simulink model "matrixmul_sysgen_cosim"  (R2017a)
settings: Solver=VariableStepAuto  StartTime=0.0  StopTime=45  RelTol=1e-3
values from neighbouring files (symbols this model uses):
  A = [1 2 8 4; 5 2 7 0; 9 10 4 2; 7 0 3 1]    [loadmatrix.m]
undefined symbols (not defined in the file or in its folder): N
libraries: xbsIndex_r4 x26, JTAGRuntimeCosim_r4 x1
settings Model: Creator=jhell  LastModifiedBy=jlh24

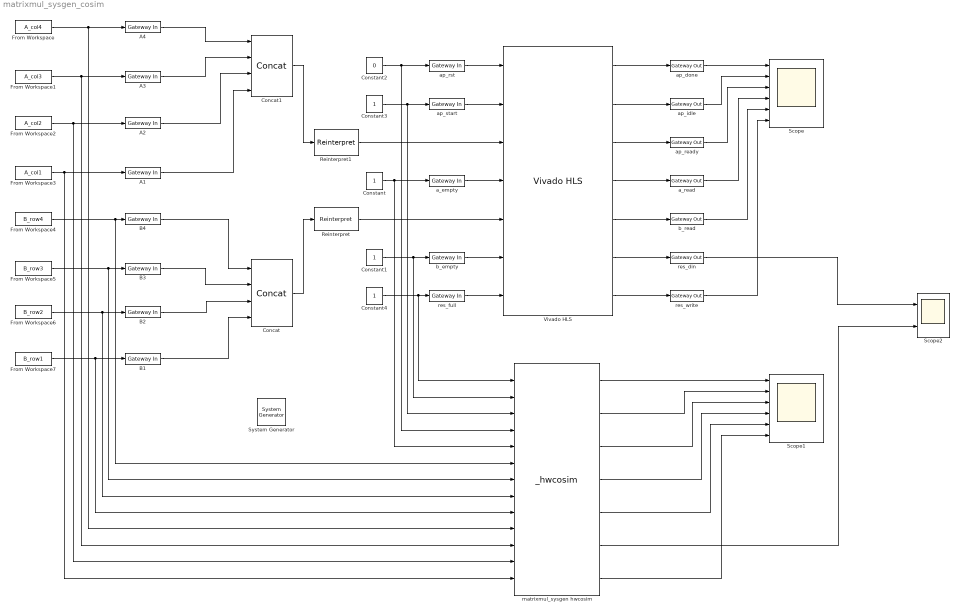
== system matrixmul_sysgen_cosim ==
  " System Generator" : xbsIndex_r4/ System Generator  Tag=genX  xilinxfamily=zynq  part=xc7z020  speed=-1  package=clg484  synthesis_tool=Vivado  clock_wrapper=Clock Enables  directory=./netlist_cosim  proj_type=Vivado  Synth_file=Vivado Synthesis Defaults  Impl_file=Vivado Implementation Defaults  testbench=off  simulink_period=1  sysclk_period=10  dcm_input_clock_period=10  incr_netlist=off  trim_vbits=Everywhere in SubSystem  dbl_ovrd=According to Block Masks  core_generation=According to Block Masks  run_coregen=off  deprecated_control=off  eval_field=0  block_type=sysgen
  A{1..4} (4 alike) : xbsIndex_r4/Gateway In  gui_display_data_type=Fixed-point  arith_type=Unsigned  n_bits=16  bin_pt=0  preci_type=Single  exp_width=8  frac_width=24  rows=1  columns=1  quantization="Round  (unbiased: +/- Inf)"  overflow=Saturate  period=1  UseAsADC=off  ADCChannel='1'  interface=None  automatic_assignment=on  address_offset=hex2dec('00')  intf_name=''  intf_description=''  default_value=0  timing_constraint=None  locs_specified=off  LOCs={}  io_standard={}  inherit_from_input=off  hdl_port=on  dbl_ovrd=off  block_type=gatewayin
  B{1..4} (4 alike) : xbsIndex_r4/Gateway In  gui_display_data_type=Fixed-point  arith_type=Unsigned  n_bits=16  bin_pt=0  preci_type=Single  exp_width=8  frac_width=24  rows=1  columns=1  quantization="Round  (unbiased: +/- Inf)"  overflow=Saturate  period=1  UseAsADC=off  ADCChannel='1'  interface=None  automatic_assignment=on  address_offset=hex2dec('00')  intf_name=''  intf_description=''  default_value=0  timing_constraint=None  locs_specified=off  LOCs={}  io_standard={}  inherit_from_input=off  hdl_port=on  dbl_ovrd=off  block_type=gatewayin
  Concat : xbsIndex_r4/Concat  num_inputs=4  dbl_ovrd=off  block_type=concat
  Concat1 : xbsIndex_r4/Concat  num_inputs=4  dbl_ovrd=off  block_type=concat
  Constant{,1,3..4} (4 alike) : Constant
  Constant2 : Constant  Value=0
  From Workspace : FromWorkspace  VariableName=A_col4  SampleTime=0  Interpolate=off  OutputAfterFinalValue=Setting to zero
  From Workspace1 : FromWorkspace  VariableName=A_col3  SampleTime=0  Interpolate=off  OutputAfterFinalValue=Setting to zero
  From Workspace2 : FromWorkspace  VariableName=A_col2  SampleTime=0  Interpolate=off  OutputAfterFinalValue=Setting to zero
  From Workspace3 : FromWorkspace  VariableName=A_col1  SampleTime=0  Interpolate=off  OutputAfterFinalValue=Setting to zero
  From Workspace4 : FromWorkspace  VariableName=B_row4  SampleTime=0  Interpolate=off  OutputAfterFinalValue=Setting to zero
  From Workspace5 : FromWorkspace  VariableName=B_row3  SampleTime=0  Interpolate=off  OutputAfterFinalValue=Setting to zero
  From Workspace6 : FromWorkspace  VariableName=B_row2  SampleTime=0  Interpolate=off  OutputAfterFinalValue=Setting to zero
  From Workspace7 : FromWorkspace  VariableName=B_row1  SampleTime=0  Interpolate=off  OutputAfterFinalValue=Setting to zero
  Reinterpret : xbsIndex_r4/Reinterpret  force_arith_type=on  arith_type="Signed  (2's comp)"  force_bin_pt=off  bin_pt=0  block_type=reinterpret
  Reinterpret1 : xbsIndex_r4/Reinterpret  force_arith_type=on  arith_type="Signed  (2's comp)"  force_bin_pt=off  bin_pt=0  block_type=reinterpret
  Scope : Scope  NumInputPorts=6
  Scope1 : Scope  NumInputPorts=6
  Scope2 : Scope  NumInputPorts=2
  Vivado HLS : xbsIndex_r4/Vivado HLS  anytable='C:/ELEC522/hellar/Project_3/matrixmul_final/matrixmul_final/solution1'  fast_sim=off  display_datatype=on  rate_propagation_method=Simulink system period  model_file_path=''  latency=1  block_type=hls
      settings: infoedit=This block allows including C,C++ and SystemC source files in System Generator for DSP designs.
  a_empty : xbsIndex_r4/Gateway In  gui_display_data_type=Boolean  arith_type=Boolean  n_bits=16  bin_pt=14  preci_type=Single  exp_width=8  frac_width=24  rows=1  columns=1  quantization="Round  (unbiased: +/- Inf)"  overflow=Saturate  period=1  UseAsADC=off  ADCChannel='1'  interface=None  automatic_assignment=on  address_offset=hex2dec('00')  intf_name=''  intf_description=''  default_value=0  timing_constraint=None  locs_specified=off  LOCs={}  io_standard={}  inherit_from_input=off  hdl_port=on  dbl_ovrd=off  block_type=gatewayin
  a_read : xbsIndex_r4/Gateway Out  inherit_from_input=off  hdl_port=on  rows=1  columns=1  UseAsDAC=off  DACChannel='1'  interface=None  automatic_assignment=on  address_offset=hex2dec('00')  intf_name=''  intf_description=''  timing_constraint=None  locs_specified=off  LOCs={}  io_standard={}  block_type=gatewayout
  ap_done : xbsIndex_r4/Gateway Out  inherit_from_input=off  hdl_port=on  rows=1  columns=1  UseAsDAC=off  DACChannel='1'  interface=None  automatic_assignment=on  address_offset=hex2dec('00')  intf_name=''  intf_description=''  timing_constraint=None  locs_specified=off  LOCs={}  io_standard={}  block_type=gatewayout
  ap_idle : xbsIndex_r4/Gateway Out  inherit_from_input=off  hdl_port=on  rows=1  columns=1  UseAsDAC=off  DACChannel='1'  interface=None  automatic_assignment=on  address_offset=hex2dec('00')  intf_name=''  intf_description=''  timing_constraint=None  locs_specified=off  LOCs={}  io_standard={}  block_type=gatewayout
  ap_ready : xbsIndex_r4/Gateway Out  inherit_from_input=off  hdl_port=on  rows=1  columns=1  UseAsDAC=off  DACChannel='1'  interface=None  automatic_assignment=on  address_offset=hex2dec('00')  intf_name=''  intf_description=''  timing_constraint=None  locs_specified=off  LOCs={}  io_standard={}  block_type=gatewayout
  ap_rst : xbsIndex_r4/Gateway In  gui_display_data_type=Boolean  arith_type=Boolean  n_bits=16  bin_pt=14  preci_type=Single  exp_width=8  frac_width=24  rows=1  columns=1  quantization="Round  (unbiased: +/- Inf)"  overflow=Saturate  period=1  UseAsADC=off  ADCChannel='1'  interface=None  automatic_assignment=on  address_offset=hex2dec('00')  intf_name=''  intf_description=''  default_value=0  timing_constraint=None  locs_specified=off  LOCs={}  io_standard={}  inherit_from_input=off  hdl_port=on  dbl_ovrd=off  block_type=gatewayin
  ap_start : xbsIndex_r4/Gateway In  gui_display_data_type=Boolean  arith_type=Boolean  n_bits=16  bin_pt=14  preci_type=Single  exp_width=8  frac_width=24  rows=1  columns=1  quantization="Round  (unbiased: +/- Inf)"  overflow=Saturate  period=1  UseAsADC=off  ADCChannel='1'  interface=None  automatic_assignment=on  address_offset=hex2dec('00')  intf_name=''  intf_description=''  default_value=0  timing_constraint=None  locs_specified=off  LOCs={}  io_standard={}  inherit_from_input=off  hdl_port=on  dbl_ovrd=off  block_type=gatewayin
  b_empty : xbsIndex_r4/Gateway In  gui_display_data_type=Boolean  arith_type=Boolean  n_bits=16  bin_pt=14  preci_type=Single  exp_width=8  frac_width=24  rows=1  columns=1  quantization="Round  (unbiased: +/- Inf)"  overflow=Saturate  period=1  UseAsADC=off  ADCChannel='1'  interface=None  automatic_assignment=on  address_offset=hex2dec('00')  intf_name=''  intf_description=''  default_value=0  timing_constraint=None  locs_specified=off  LOCs={}  io_standard={}  inherit_from_input=off  hdl_port=on  dbl_ovrd=off  block_type=gatewayin
  b_read : xbsIndex_r4/Gateway Out  inherit_from_input=off  hdl_port=on  rows=1  columns=1  UseAsDAC=off  DACChannel='1'  interface=None  automatic_assignment=on  address_offset=hex2dec('00')  intf_name=''  intf_description=''  timing_constraint=None  locs_specified=off  LOCs={}  io_standard={}  block_type=gatewayout
  matrixmul_sysgen hwcosim : JTAGRuntimeCosim_r4/_hwcosim  clkSrc=Single Stepped  hasCombinationalPath=on  bitfileName=C:\ELEC522\hellar\Project_3\matrixmul_final\netlist_cosim\matrixmul_sysgen.bit  skipConfig=off  dispPartInfo=off  useZynqReconfigScript=on  cable=Auto Detect  speed=N/A  cablePort=N/A  cableLocation=Local  shareCable=off  design_xtable=|  engineDll=JTAGCosimEngine.dll  cableWaitTime=10  bscanPos=-1  IRLengths=[]  useWaitBox=1  hasBufgmux=on  Scheme=Cosim  useCmdProc=1  hasProc=0  useImpact=0  printLogFile=0  userChain=2  block_type=jtagcosim
      | {
      |     'clkWrapper' => 'matrixmul_sysgen',
      |     'burstMode' => false,
      |     'burstFifoDepth' => '1024',
      |     'shared_memories' => {},
      |     'clocksGcd' => 1,
      |     'device' => {
      |       'family' => 'zynq',
      |       'part' => 'xc7z020',
      |       'package' => 'clg484',
      |       'speed' => '-1',
      |     },
      |     'ports' => {
      |       'res_full' => {
      |         'direction' => 'in',
      |         'width' => 1,
      |         'name' => 'res_full',
      |         'period' => 1,
      |         'icon_text' => 'res_full',
      |         'type' => 'Bool',
      |         'arithmetic_type' => 'xlUnsigned',
      |         'dat_file' => 'matrixmul_sysgen_res_full.dat',
      |         'bin_pt' => 0,
      |         'addr_offset' => 0,
      |         'bd_port_index' => 0,
      |       },
      |       'b_empty' => {
      |         'direction' => 'in',
      |         'width' => 1,
      |         'name' => 'b_empty',
      |         'period' => 1,
      |         'icon_text' => 'b_empty',
      |         'type' => 'Bool',
      |         'arithmetic_type' => 'xlUnsigned',
      |         'dat_file' => 'matrixmul_sysgen_b_empty.dat',
      |         'bin_pt' => 0,
      |         'addr_offset' => 4,
      |         'bd_port_index' => 1,
      |       },
      |       'ap_start' => {
      |         'direction' => 'in',
      |         'width' => 1,
      |         'name' => 'ap_start',
      |         'period' => 1,
      |         'icon_text' => 'ap_start',
      |         'type' => 'Bool',
      |         'arithmetic_type' => 'xlUnsigned',
      |         'dat_file' => 'matrixmul_sysgen_ap_start.dat',
      |         'bin_pt' => 0,
      |         'addr_offset' => 8,
      |         'bd_port_index' => 2,
      |       },
      |       'ap_rst' => {
      |         'direction' => 'in',
      |         'width' => 1,
      |         'name' => 'ap_rst',
      |         'period' => 1,
      |         'icon_text' => 'ap_rst',
      |         'type' => 'Bool',
      |         'arithmetic_type' => 'xlUnsigned',
      |         'dat_file' => 'matrixmul_sysgen_ap_rst.dat',
      |         'bin_pt' => 0,
      |         'addr_offset' => 12,
      |         'bd_port_index' => 3,
      |       },
      |       'a_empty' => {
      |         'direction' => 'in',
      |         'width' => 1,
      |         'name' => 'a_empty',
      |         'period' => 1,
      |         'icon_text' => 'a_empty',
      |         'type' => 'Bool',
      |         'arithmetic_type' => 'xlUnsigned',
      |         'dat_file' => 'matrixmul_sysgen_a_empty.dat',
      |         'bin_pt' => 0,
      |         'addr_offset' => 16,
      |         'bd_port_index' => 4,
      |       },
      |       'b4' => {
      |         'direction' => 'in',
      |         'width' => 16,
      |         'name' => 'b4',
      |         'period' => 1,
      |         'icon_text' => 'B4',
      |         'type' => 'UFix_16_0',
      |         'arithmetic_type' => 'xlUnsigned',
      |         'dat_file' => 'matrixmul_sysgen_b4.dat',
      |         'bin_pt' => 0,
      |         'addr_offset' => 20,
      |         'bd_port_index' => 5,
      |       },
      |       'b3' => {
      |         'direction' => 'in',
      |         'width' => 16,
      |         'name' => 'b3',
      |         'period' => 1,
      |         'icon_text' => 'B3',
      |         'type' => 'UFix_16_0',
      |         'arithmetic_type' => 'xlUnsigned',
      |         'dat_file' => 'matrixmul_sysgen_b3.dat',
      |         'bin_pt' => 0,
      |         'addr_offset' => 24,
      |         'bd_port_index' => 6,
      |       },
      |       'b2' => {
      |         'direction' => 'in',
      |         'width' => 16,
      |         'name' => 'b2',
      |         'period' => 1,
      |         'icon_text' => 'B2',
      |         'type' => 'UFix_16_0',
      |         'arithmetic_type' => 'xlUnsigned',
      |         'dat_file' => 'matrixmul_sysgen_b2.dat',
      |         'bin_pt' => 0,
      |         'addr_offset' => 28,
      |         'bd_port_index' => 7,
      |       },
      |       'b1' => {
      |         'direction' => 'in',
      |         'width' => 16,
      |         'name' => 'b1',
      |         'period' => 1,
      |         'icon_text' => 'B1',
      |         'type' => 'UFix_16_0',
      |         'arithmetic_type' => 'xlUnsigned',
      |         'dat_file' => 'matrixmul_sysgen_b1.dat',
      |         'bin_pt' => 0,
      |         'addr_offset' => 32,
      |         'bd_port_index' => 8,
      |       },
      |       'a4' => {
      |         'direction' => 'in',
      |         'width' => 16,
      |         'name' => 'a4',
      |         'period' => 1,
      |         'icon_text' => 'A4',
      |         'type' => 'UFix_16_0',
      |         'arithmetic_type' => 'xlUnsigned',
      |         'dat_file' => 'matrixmul_sysgen_a4.dat',
      |         'bin_pt' => 0,
      |         'addr_offset' => 36,
      |         'bd_port_index' => 9,
      |       },
      |       'a3' => {
      |         'direction' => 'in',
      |         'width' => 16,
      |         'name' => 'a3',
      |         'period' => 1,
      |         'icon_text' => 'A3',
      |         'type' => 'UFix_16_0',
      |         'arithmetic_type' => 'xlUnsigned',
      |         'dat_file' => 'matrixmul_sysgen_a3.dat',
      |         'bin_pt' => 0,
      |         'addr_offset' => 40,
      |         'bd_port_index' => 10,
      |       },
      |       'a2' => {
      |         'direction' => 'in',
      |         'width' => 16,
      |         'name' => 'a2',
      |         'period' => 1,
      |         'icon_text' => 'A2',
      |         'type' => 'UFix_16_0',
      |         'arithmetic_type' => 'xlUnsigned',
      |         'dat_file' => 'matrixmul_sysgen_a2.dat',
      |         'bin_pt' => 0,
      |         'addr_offset' => 44,
      |         'bd_port_index' => 11,
      |       },
      |       'a1' => {
      |         'direction' => 'in',
      |         'width' => 16,
      |         'name' => 'a1',
      |         'period' => 1,
      |         'icon_text' => 'A1',
      |         'type' => 'UFix_16_0',
      |         'arithmetic_type' => 'xlUnsigned',
      |         'dat_file' => 'matrixmul_sysgen_a1.dat',
      |         'bin_pt' => 0,
      |         'addr_offset' => 48,
      |         'bd_port_index' => 12,
      |       },
      |       'a_read' => {
      |         'direction' => 'out',
      |         'width' => 1,
      |         'name' => 'a_read',
      |         'period' => 1,
      |         'icon_text' => 'a_read',
      |         'type' => 'Bool',
      |         'arithmetic_type' => 'xlUnsigned',
      |         'dat_file' => 'matrixmul_sysgen_a_read.dat',
      |         'bin_pt' => 0,
      |         'addr_offset' => 52,
      |         'bd_port_index' => 0,
      |       },
      |       'ap_done' => {
      |         'direction' => 'out',
      |         'width' => 1,
      |         'name' => 'ap_done',
      |         'period' => 1,
      |         'icon_text' => 'ap_done',
      |         'type' => 'Bool',
      |         'arithmetic_type' => 'xlUnsigned',
      |         'dat_file' => 'matrixmul_sysgen_ap_done.dat',
      |         'bin_pt' => 0,
      |         'addr_offset' => 56,
      |         'bd_port_index' => 1,
      |       },
      |       'ap_idle' => {
      |         'direction' => 'out',
      |         'width' => 1,
      |         'name' => 'ap_idle',
      |         'period' => 1,
      |         'icon_text' => 'ap_idle',
      |         'type' => 'Bool',
      |         'arithmetic_type' => 'xlUnsigned',
      |         'dat_file' => 'matrixmul_sysgen_ap_idle.dat',
      |         'bin_pt' => 0,
      |         'addr_offset' => 60,
      |         'bd_port_index' => 2,
      |       },
      |       'ap_ready' => {
      |         'direction' => 'out',
      |         'width' => 1,
      |         'name' => 'ap_ready',
      |         'period' => 1,
      |         'icon_text' => 'ap_ready',
      |         'type' => 'Bool',
      |         'arithmetic_type' => 'xlUnsigned',
      |         'dat_file' => 'matrixmul_sysgen_ap_ready.dat',
      |         'bin_pt' => 0,
      |         'addr_offset' => 64,
      |         'bd_port_index' => 3,
      |       },
      |       'b_read' => {
      |         'direction' => 'out',
      |         'width' => 1,
      |         'name' => 'b_read',
      |         'period' => 1,
      |         'icon_text' => 'b_read',
      |         'type' => 'Bool',
      |         'arithmetic_type' => 'xlUnsigned',
      |         'dat_file' => 'matrixmul_sysgen_b_read.dat',
      |         'bin_pt' => 0,
      |         'addr_offset' => 68,
      |         'bd_port_index' => 4,
      |       },
      |       'res_din' => {
      |         'direction' => 'out',
      |         'width' => 16,
      |         'name' => 'res_din',
      |         'period' => 1,
      |         'icon_text' => 'res_din',
      |         'type' => 'Fix_16_0',
      |         'arithmetic_type' => 'xlSigned',
      |         'dat_file' => 'matrixmul_sysgen_res_din.dat',
      |         'bin_pt' => 0,
      |         'addr_offset' => 72,
      |         'bd_port_index' => 5,
      |       },
      |       'res_write' => {
      |         'direction' => 'out',
      |         'width' => 1,
      |         'name' => 'res_write',
      |         'period' => 1,
      |         'icon_text' => 'res_write',
      |         'type' => 'Bool',
      |         'arithmetic_type' => 'xlUnsigned',
      |         'dat_file' => 'matrixmul_sysgen_res_write.dat',
      |         'bin_pt' => 0,
      |         'addr_offset' => 76,
      |         'bd_port_index' => 6,
      |       },
      |     },
      |   }
  res_din : xbsIndex_r4/Gateway Out  inherit_from_input=off  hdl_port=on  rows=1  columns=1  UseAsDAC=off  DACChannel='1'  interface=None  automatic_assignment=on  address_offset=hex2dec('00')  intf_name=''  intf_description=''  timing_constraint=None  locs_specified=off  LOCs={}  io_standard={}  block_type=gatewayout
  res_full : xbsIndex_r4/Gateway In  gui_display_data_type=Boolean  arith_type=Boolean  n_bits=16  bin_pt=14  preci_type=Single  exp_width=8  frac_width=24  rows=1  columns=1  quantization="Round  (unbiased: +/- Inf)"  overflow=Saturate  period=1  UseAsADC=off  ADCChannel='1'  interface=None  automatic_assignment=on  address_offset=hex2dec('00')  intf_name=''  intf_description=''  default_value=0  timing_constraint=None  locs_specified=off  LOCs={}  io_standard={}  inherit_from_input=off  hdl_port=on  dbl_ovrd=off  block_type=gatewayin
  res_write : xbsIndex_r4/Gateway Out  inherit_from_input=off  hdl_port=on  rows=1  columns=1  UseAsDAC=off  DACChannel='1'  interface=None  automatic_assignment=on  address_offset=hex2dec('00')  intf_name=''  intf_description=''  timing_constraint=None  locs_specified=off  LOCs={}  io_standard={}  block_type=gatewayout
  wires:
  ap_start/1 -> Vivado HLS/2
  a_empty/1 -> Vivado HLS/4
  Constant3/1 -> matrixmul_sysgen hwcosim/3, ap_start/1
  Constant/1 -> matrixmul_sysgen hwcosim/5, a_empty/1
  Constant1/1 -> matrixmul_sysgen hwcosim/2, b_empty/1
  b_empty/1 -> Vivado HLS/6
  res_full/1 -> Vivado HLS/7
  Reinterpret/1 -> Vivado HLS/5
  Concat/1 -> Reinterpret/1
  Concat1/1 -> Reinterpret1/1
  A4/1 -> Concat1/1
  A3/1 -> Concat1/2
  A2/1 -> Concat1/3
  A1/1 -> Concat1/4
  B4/1 -> Concat/1
  B3/1 -> Concat/2
  B2/1 -> Concat/3
  B1/1 -> Concat/4
  From Workspace/1 -> matrixmul_sysgen hwcosim/10, A4/1
  From Workspace1/1 -> matrixmul_sysgen hwcosim/11, A3/1
  From Workspace2/1 -> matrixmul_sysgen hwcosim/12, A2/1
  From Workspace3/1 -> matrixmul_sysgen hwcosim/13, A1/1
  From Workspace4/1 -> matrixmul_sysgen hwcosim/6, B4/1
  From Workspace5/1 -> matrixmul_sysgen hwcosim/7, B3/1
  From Workspace6/1 -> matrixmul_sysgen hwcosim/8, B2/1
  From Workspace7/1 -> matrixmul_sysgen hwcosim/9, B1/1
  ap_rst/1 -> Vivado HLS/1
  Constant2/1 -> matrixmul_sysgen hwcosim/4, ap_rst/1
  Reinterpret1/1 -> Vivado HLS/3
  res_din/1 -> Scope2/1
  Vivado HLS/1 -> ap_done/1
  Vivado HLS/2 -> ap_idle/1
  Vivado HLS/3 -> ap_ready/1
  Vivado HLS/7 -> res_write/1
  Vivado HLS/6 -> res_din/1
  Vivado HLS/5 -> b_read/1
  Vivado HLS/4 -> a_read/1
  ap_done/1 -> Scope/1
  ap_idle/1 -> Scope/2
  ap_ready/1 -> Scope/3
  a_read/1 -> Scope/4
  b_read/1 -> Scope/5
  res_write/1 -> Scope/6
  Constant4/1 -> matrixmul_sysgen hwcosim/1, res_full/1
  matrixmul_sysgen hwcosim/2 -> Scope1/2
  matrixmul_sysgen hwcosim/1 -> Scope1/1
  matrixmul_sysgen hwcosim/3 -> Scope1/3
  matrixmul_sysgen hwcosim/4 -> Scope1/4
  matrixmul_sysgen hwcosim/5 -> Scope1/5
  matrixmul_sysgen hwcosim/7 -> Scope1/6
  matrixmul_sysgen hwcosim/6 -> Scope2/2
